simulink model "Thermal_Energy"  (Simulink 9.0)
settings: Solver=ode3  StartTime=0.0  StopTime=200100  FixedStep=T  RelTol=1e-3  EnableMultiTasking=on
values from neighbouring files (symbols this model uses):
  T = 0.01    [APRBS_Anregung_APRBS.m]    (also in ini_gdnn.m)
settings Model: Creator=Ussaema  LastModifiedBy=Ussaema
settings DataIOCC: LimitDataPoints=on  SignalLoggingSaveFormat=ModelDataLogs
settings OptimizationCC: InitFltsAndDblsToZero=on
settings DebuggingCC: SaveWithParameterizedLinksMsg=none  SignalResolutionControl=TryResolveAllWithWarning  SolverPrmCheckMsg=warning  MultiTaskDSMMsg=warning  MultiTaskCondExecSysMsg=none  FcnCallInpInsideContextMsg=warning  StrictBusMsg=Warning
settings GRTTargetCC: TargetFcnLib=ansi_tfl_tmw.mat  CombineOutputUpdateFcns=off  GRTInterface=on

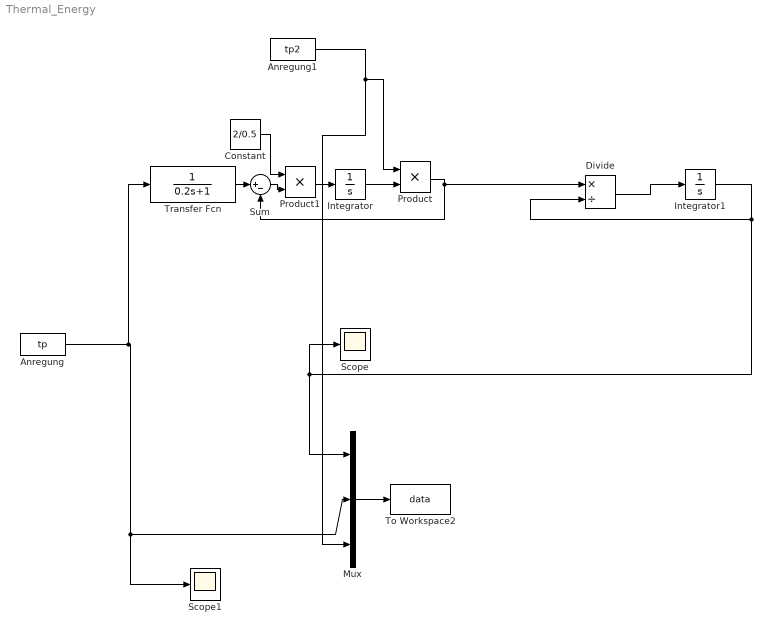
== system Thermal_Energy ==
  Anregung : FromWorkspace  VariableName=tp  SampleTime=T  Interpolate=off  OutputAfterFinalValue=Cyclic repetition
  Anregung1 : FromWorkspace  VariableName=tp2  SampleTime=T  Interpolate=off  OutputAfterFinalValue=Cyclic repetition
  Constant : Constant  Value=2/0.5
  Divide : Product  Inputs=*/
  Integrator : Integrator
  Integrator1 : Integrator  InitialCondition=0.1
  Mux : Mux  Inputs=3
  Product : Product
  Product1 : Product
  Scope : Scope
  Scope1 : Scope
  Sum : Sum  Inputs=|+-
  To Workspace2 : ToWorkspace  VariableName=data  SaveFormat=Structure With Time  SampleTime=-1
  Transfer Fcn : TransferFcn  Denominator=[0.2 1]
  wires:
  Mux/1 -> To Workspace2/1
  Transfer Fcn/1 -> Sum/1
  Anregung/1 -> Transfer Fcn/1, Scope1/1, Mux/2
  Integrator1/1 -> Mux/1, Scope/1, Divide/2
  Integrator/1 -> Product/2
  Anregung1/1 -> Mux/3, Product/1
  Product1/1 -> Integrator/1
  Sum/1 -> Product1/2
  Divide/1 -> Integrator1/1
  Constant/1 -> Product1/1
  Product/1 -> Divide/1, Sum/2
